simulink model "turbojetmatch"  (R2018a)
settings: Solver=VariableStepAuto  StartTime=0.0  StopTime=0  RelTol=1e-3
libraries: motorlib x7
settings Model: Creator=mairon  LastModifiedBy=mairon

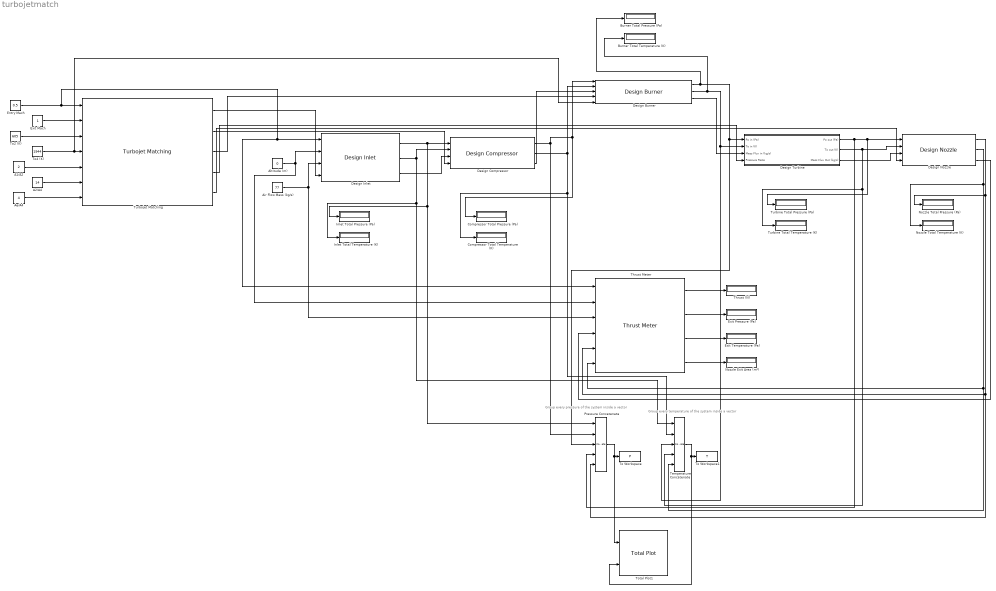
== system turbojetmatch ==
  note: Group every temperature of the system inside a vector
  note: Group every pressure of the system inside a vector
  A1/A2 : Constant  Value=2
  A2/A4 : Constant  Value=14
  Ae/A4 : Constant  Value=4
  Air Flow Mass (kg/s) : Constant  Value=77
  Altitude (m) : Constant  Value=0
  Burner Total Pressure (Pa) : Display
  Burner Total Temperature (K) : Display
  Compressor Total Pressure (Pa) : Display
  Compressor Total Temperature (K) : Display
  Design Burner : motorlib/Design Burner
      settings: SourceProductName=Aeronautic Motor
  Design Compressor : motorlib/Design Compressor
      settings: SourceProductName=Aeronautic Motor
  Design Inlet : motorlib/Design Inlet
      settings: SourceProductName=Aeronautic Motor
  Design Nozzle : motorlib/Design Nozzle
      settings: SourceProductName=Aeronautic Motor
  Design Turbine : Subsystem
  Entry Mach : Constant  Value=0.5
  Exit Mach : Constant
  Exit Pressure (Pa) : Display
  Exit Temperature (Pa) : Display
  Inlet Total Pressure (Pa) : Display
  Inlet Total Temperature (K) : Display
  Nozzle Exit Area (m²) : Display
  "Nozzle Total Pressure (Pa) " : Display
  Nozzle Total Temperature (K) : Display
  Pressure Concatenate : Concatenate  NumInputs=5
  Temperature Concatenate : Concatenate  NumInputs=5
  Thrust (N) : Display
  Thrust Meter : motorlib/Thrust Meter
      settings: SourceProductName=Aeronautic Motor
  To Workspace : ToWorkspace  VariableName=P  SaveFormat=Timeseries  SampleTime=-1
  To Workspace1 : ToWorkspace  VariableName=T  SaveFormat=Timeseries  SampleTime=-1
  To2 (K) : Constant  Value=605
  To4 (K) : Constant  Value=1944
  Total Plot1 : motorlib/Total Plot
      settings: SourceProductName=Aeronautic Motor
  Turbine Total Pressure (Pa) : Display
  Turbine Total Temperature (K) : Display
  Turbojet Matching : motorlib/Turbojet Matching
      settings: SourceProductName=Aeronautic Motor
  wires:
  Entry Mach/1 -> Design Inlet/1, Thrust Meter/1, Turbojet Matching/1
  Altitude (m)/1 -> Design Inlet/2, Thrust Meter/2
  Design Inlet/1 -> Design Compressor/1, Inlet Total Pressure (Pa)/1, Pressure Concatenate/1
  Air Flow Mass (kg/s)/1 -> Design Inlet/3, Thrust Meter/3
  Design Nozzle/1 -> Pressure Concatenate/5, Thrust Meter/5, "Nozzle Total Pressure (Pa) "/1
  Design Nozzle/2 -> Temperature Concatenate/5, Thrust Meter/6, Nozzle Total Temperature (K)/1
  Design Inlet/2 -> Design Compressor/2, Temperature Concatenate/1, Inlet Total Temperature (K)/1
  Design Inlet/3 -> Design Compressor/3
  Design Compressor/1 -> Design Burner/1, Compressor Total Pressure (Pa)/1, Pressure Concatenate/2
  Design Compressor/2 -> Design Burner/2, Temperature Concatenate/2, Compressor Total Temperature (K)/1
  Design Compressor/3 -> Design Burner/3
  Design Burner/1 -> Design Turbine/1(Po in (Pa)), Pressure Concatenate/3, Burner Total Pressure (Pa)/1
  Design Burner/2 -> Design Turbine/2(To in (K)), Temperature Concatenate/3, Burner Total Temperature (K)/1
  Design Burner/3 -> Design Turbine/3(Mass Flux in (kg/s))
  Design Turbine/1(Po out (Pa)) -> Pressure Concatenate/4, Design Nozzle/1, Turbine Total Pressure (Pa)/1
  Design Turbine/3(Mass Flux Out (kg/s)) -> Design Nozzle/3
  Design Turbine/2(To out (K)) -> Temperature Concatenate/4, Turbine Total Temperature (K)/1, Design Nozzle/2
  Design Nozzle/3 -> Thrust Meter/4
  Thrust Meter/1 -> Thrust (N)/1
  Thrust Meter/2 -> Exit Pressure (Pa)/1
  Thrust Meter/3 -> Exit Temperature (Pa)/1
  Thrust Meter/4 -> Nozzle Exit Area (m²)/1
  Pressure Concatenate/1 -> Total Plot1/1, To Workspace/1
  Temperature Concatenate/1 -> Total Plot1/2, To Workspace1/1
  Exit Mach/1 -> Turbojet Matching/2
  To2 (K)/1 -> Turbojet Matching/3
  To4 (K)/1 -> Design Burner/5, Turbojet Matching/4
  A1/A2/1 -> Turbojet Matching/5
  A2/A4/1 -> Turbojet Matching/6
  Ae/A4/1 -> Turbojet Matching/7
  Turbojet Matching/1 -> Design Inlet/4
  Turbojet Matching/2 -> Design Compressor/4
  Turbojet Matching/3 -> Design Burner/4
  Turbojet Matching/4 -> Design Turbine/4(Pressure Ratio)
  Turbojet Matching/5 -> Design Nozzle/4

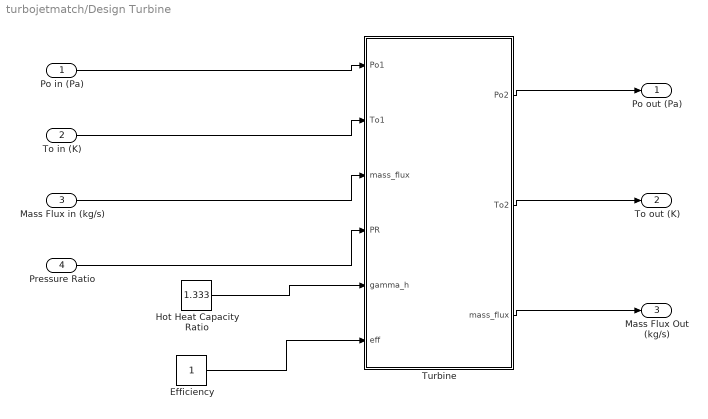
== system turbojetmatch/Design Turbine ==
  Po in (Pa) : Inport
  To in (K) : Inport  Port=2
  Mass Flux in (kg/s) : Inport  Port=3
  Pressure Ratio : Inport  Port=4
  Efficiency : Constant
  Hot Heat Capacity Ratio : Constant  Value=1.333
  Turbine : MATLAB Function  TreatAsAtomicUnit=on
  Po out (Pa) : Outport
  To out (K) : Outport  Port=2
  Mass Flux Out (kg/s) : Outport  Port=3
  wires:
  Turbine/2(To2) -> To out (K)/1
  To in (K)/1 -> Turbine/2(To1)
  Pressure Ratio/1 -> Turbine/4(PR)
  Turbine/1(Po2) -> Po out (Pa)/1
  Hot Heat Capacity Ratio/1 -> Turbine/5(gamma_h)
  Turbine/3(mass_flux) -> Mass Flux Out (kg/s)/1
  Po in (Pa)/1 -> Turbine/1(Po1)
  Mass Flux in (kg/s)/1 -> Turbine/3("mass_flux ")
  Efficiency/1 -> Turbine/6(eff)

== matlab function turbojetmatch/Design Turbine/Turbine ==
  data: Po1 input; To1 input; mass_flux input; PR input; Po2 output; To2 output; gamma_h input; mass_flux output; eff input
function [Po2,To2,mass_flux]  = Turbine(Po1,To1,mass_flux,PR,gamma_h,eff)   
    Po2 = PR*Po1;   % total pressure   
    To2s = PR^((gamma_h-1)/gamma_h) * To1
    To2 = (To2s - To1)*eff + To1
